simulink model "Progetto_a1_simulink_lineare"  (R2022b)
settings: Solver=VariableStepAuto  StartTime=0.0  StopTime=10  RelTol=1e-3
values from neighbouring files (symbols this model uses):
  DD_ampiezza = 0.3    [Progetto_a1.m]
  DD_frequenza = 0.025    [Progetto_a1.m]
  denG = deG{1}    [Progetto_a1.m]
  denR = deR{1}    [Progetto_a1.m]
  NN_ampiezza = 0.2    [Progetto_a1.m]
  NN_frequenza = 1e3    (= 1000)    [Progetto_a1.m]
  numG = nuG{1}    [Progetto_a1.m]
  numR = nuR{1}    [Progetto_a1.m]
  WW_check = -2    [Progetto_a1.m]
  x = [1,2,3,4]    [Progetto_a1.m]
settings Model: Creator=anton  LastModifiedBy=anton

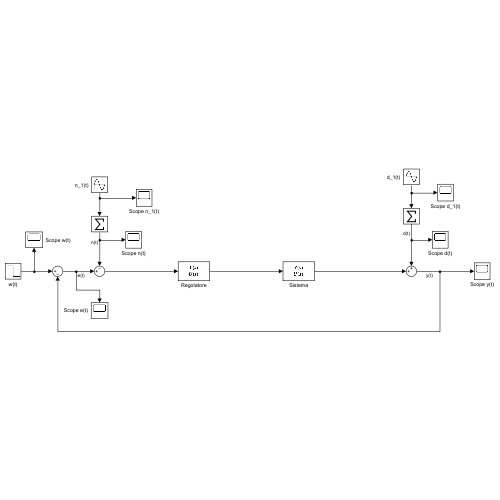
[thumbnail: Simulink's stored preview of the top-level diagram]
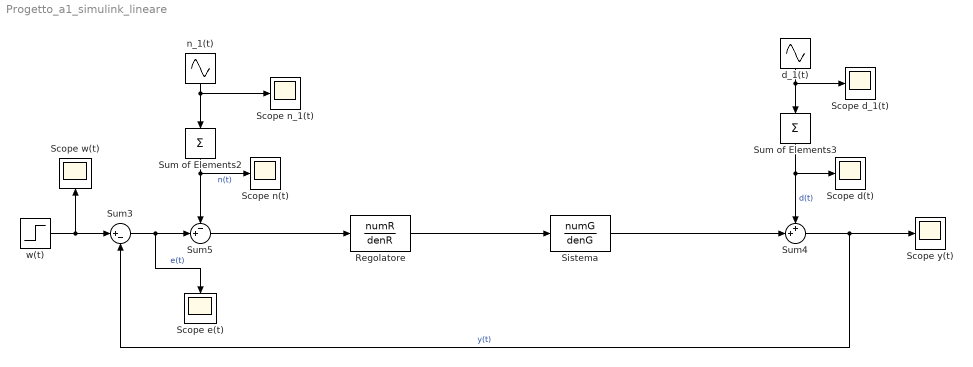
== system Progetto_a1_simulink_lineare ==
  Regolatore : TransferFcn  Numerator=numR  Denominator=denR
  Scope d(t) : Scope
  Scope d_1(t) : Scope
  Scope e(t) : Scope
  Scope n(t) : Scope
  Scope n_1(t) : Scope
  Scope w(t) : Scope
  Scope y(t) : Scope
  Sistema : TransferFcn  Numerator=numG  Denominator=denG
  Sum of Elements2 : Sum  Inputs=+  CollapseDim=4
  Sum of Elements3 : Sum  Inputs=+  CollapseDim=4
  Sum3 : Sum  Inputs=|+-
  Sum4 : Sum  Inputs=++|
  Sum5 : Sum  Inputs=-+|
  d_1(t) : Sin  Amplitude=DD_ampiezza  Frequency=DD_frequenza*x  SampleTime=0
  n_1(t) : Sin  Amplitude=NN_ampiezza  Frequency=NN_frequenza*x  SampleTime=0
  w(t) : Step  Time=0  After=WW_check  SampleTime=0
  wires:
  Regolatore/1 -> Sistema/1
  Sum of Elements2/1 -> Sum5/1, Scope n(t)/1  "n(t)"
  Sum5/1 -> Regolatore/1
  n_1(t)/1 -> Sum of Elements2/1, Scope n_1(t)/1
  Sum3/1 -> Scope e(t)/1, Sum5/2  "e(t)"
  w(t)/1 -> Scope w(t)/1, Sum3/1
  Sum4/1 -> Scope y(t)/1, Sum3/2  "y(t)"
  d_1(t)/1 -> Sum of Elements3/1, Scope d_1(t)/1
  Sum of Elements3/1 -> Sum4/1, Scope d(t)/1  "d(t)"
  Sistema/1 -> Sum4/2
